simulink model "IEEE39_IBR_FrequencyControl_Primary_2022b"  (R2022b)
settings: Solver=VariableStepAuto  StartTime=0.0  StopTime=30  RelTol=1e-3
InitFcn:
  | IEEE39data_FrencyControl_primary;
undefined symbols (not defined in the file): Fref, IBR_data, line, Sbase, t_start_disturbance, Vbase
libraries: spsThreePhaseVIMeasurementLib x61, spsThreePhasePISectionLineLib x34, spsControlledVoltageSourceLib x33, spsabctodq0Lib x33, powerlib_extras x27, spsPLL3phLib x26, spsGroundLib x22, spsThreePhaseSeriesRLCBranchLib x22, spsThreePhaseParallelRLCLoadLib x20, slpidlib x14, spsMeanLib x11, spsdq0toabcLib x11
(part 3 of 5)

== system IEEE39_IBR_FrequencyControl_Primary_2022b/GFM4/PV_PQ3 ==
  Pref : Inport
  Vref_LL : Inport  Port=2
  Fref : Inport  Port=3
  Initial_phase : Inport  Port=4
  3-phase Instantaneous Active & Reactive Power4 : powerlib_extras/Measurements/3-phase  Instantaneous  Active & Reactive Power
  Controlled Voltage Source : spsControlledVoltageSourceLib/Controlled Voltage Source  Initialize=on  Source_Type=DC  Amplitude=0  Phase=0  Frequency=60  Measurements=None
  Controlled Voltage Source1 : spsControlledVoltageSourceLib/Controlled Voltage Source  Initialize=on  Source_Type=DC  Amplitude=0  Phase=-120  Frequency=60  Measurements=None
  Controlled Voltage Source3 : spsControlledVoltageSourceLib/Controlled Voltage Source  Initialize=on  Source_Type=DC  Amplitude=0  Phase=120  Frequency=60  Measurements=None
  Demux : Demux  Outputs=2
  Freq_Droop : Subsystem
  Ground : spsGroundLib/Ground  LConnTagsString=a
  Ground1 : spsGroundLib/Ground  LConnTagsString=a
  L : spsThreePhaseSeriesRLCBranchLib/Three-Phase Series RLC Branch  LConnTagsString=A|B|C  RConnTagsString=A|B|C  BranchType=L  Resistance=1  Inductance=0.01  Capacitance=1.0  Measurements=None
  Mean : spsMeanLib/Mean  Freq=60  Vinit=0  Ts=5e-4
  Three-Phase Series RLC Branch : spsThreePhaseSeriesRLCBranchLib/Three-Phase Series RLC Branch  LConnTagsString=A|B|C  RConnTagsString=A|B|C  BranchType=C  Resistance=0  Inductance=1e-3  Capacitance=1e-6  Measurements=None
  Three-Phase V-I Measurement : spsThreePhaseVIMeasurementLib/Three-Phase V-I Measurement  VoltageMeasurement=phase-to-ground  SetLabelV=off  LabelV=Vabc  Vpu=off  VpuLL=off  CurrentMeasurement=yes  SetLabelI=off  LabelI=Iabc  Ipu=off  Pbase=1e5  Vbase=380  OutputType=Complex  PhasorSimulation=off  PSBequivalent=0
  Three-Phase V-I Measurement4 : spsThreePhaseVIMeasurementLib/Three-Phase V-I Measurement  VoltageMeasurement=no  SetLabelV=off  LabelV=u  Vpu=off  VpuLL=off  CurrentMeasurement=yes  SetLabelI=off  LabelI=iFabcp3  Ipu=off  Pbase=100e6  Vbase=500e3  OutputType=Complex  PhasorSimulation=off  PSBequivalent=0
  Unit Delay : UnitDelay  SampleTime=-1  HasFrameUpgradeWarning=on
  Unit Delay1 : UnitDelay  SampleTime=-1  HasFrameUpgradeWarning=on
  Unit Delay2 : UnitDelay  SampleTime=-1  HasFrameUpgradeWarning=on
  V/F : Subsystem
  PV_BatteryA : PMIOPort  Side=Right
  PV_BatteryB : PMIOPort  Port=2  Side=Right
  PV_BatteryC : PMIOPort  Port=3  Side=Right
  tag scope: P_GFM7=global
  wires:
  Three-Phase V-I Measurement/1 -> 3-phase Instantaneous Active & Reactive Power4/1, V/F/1(vabcb)
  Three-Phase V-I Measurement/2 -> V/F/2(iabcb), 3-phase Instantaneous Active & Reactive Power4/2
  Mean/1 -> Demux/1
  3-phase Instantaneous Active & Reactive Power4/1 -> Mean/1
  Pref/1 -> Freq_Droop/1(Pref)
  Fref/1 -> Freq_Droop/2(Fref)
  [P_meas] -> Freq_Droop/3(Pmeans)
  Freq_Droop/1(fset) -> V/F/5(f)
  Vref_LL/1 -> V/F/4(Vref_LL)
  Initial_phase/1 -> V/F/6(Init_Phase_degree)
  Unit Delay/1 -> Controlled Voltage Source/1
  V/F/1(Va) -> Unit Delay/1
  Unit Delay1/1 -> Controlled Voltage Source1/1
  V/F/2(Vb) -> Unit Delay1/1
  Unit Delay2/1 -> Controlled Voltage Source3/1
  V/F/3(Vc) -> Unit Delay2/1
  Demux/1 -> [P_meas], [P_GFM7]
  Three-Phase V-I Measurement4/1 -> V/F/3(iFabcb)
  connections:
  Three-Phase V-I Measurement/RConn2 -- PV_BatteryB/RConn1
  Three-Phase V-I Measurement/LConn2 -- Three-Phase Series RLC Branch/LConn2 -- L/RConn2
  Three-Phase V-I Measurement4/LConn2 -- Controlled Voltage Source1/RConn1
  Controlled Voltage Source/RConn1 -- Three-Phase V-I Measurement4/LConn1
  Three-Phase V-I Measurement4/LConn3 -- Controlled Voltage Source3/RConn1
  Three-Phase V-I Measurement/LConn3 -- Three-Phase Series RLC Branch/LConn3 -- L/RConn3
  Three-Phase V-I Measurement/RConn3 -- PV_BatteryC/RConn1
  Three-Phase V-I Measurement/RConn1 -- PV_BatteryA/RConn1
  Three-Phase V-I Measurement4/RConn1 -- L/LConn1
  Three-Phase V-I Measurement4/RConn2 -- L/LConn2
  Three-Phase V-I Measurement4/RConn3 -- L/LConn3
  Three-Phase Series RLC Branch/RConn1 -- Ground1/LConn1 -- Three-Phase Series RLC Branch/RConn2 -- Three-Phase Series RLC Branch/RConn3
  Controlled Voltage Source/LConn1 -- Controlled Voltage Source3/LConn1 -- Controlled Voltage Source1/LConn1 -- Ground/LConn1
  Three-Phase V-I Measurement/LConn1 -- Three-Phase Series RLC Branch/LConn1 -- L/RConn1

== system IEEE39_IBR_FrequencyControl_Primary_2022b/PV/PV_PQ3 ==
  Pref : Inport
  Qref : Inport  Port=2
  3-phase Instantaneous Active & Reactive Power4 : powerlib_extras/Measurements/3-phase  Instantaneous  Active & Reactive Power
  Controlled Voltage Source : spsControlledVoltageSourceLib/Controlled Voltage Source  Initialize=on  Source_Type=AC  Amplitude=391.87  Phase=0  Frequency=60  Measurements=None
  Controlled Voltage Source1 : spsControlledVoltageSourceLib/Controlled Voltage Source  Initialize=on  Source_Type=AC  Amplitude=391.87  Phase=-120  Frequency=60  Measurements=None
  Controlled Voltage Source3 : spsControlledVoltageSourceLib/Controlled Voltage Source  Initialize=on  Source_Type=AC  Amplitude=391.87  Phase=120  Frequency=60  Measurements=None
  Demux : Demux  Outputs=2
  Ground : spsGroundLib/Ground  LConnTagsString=a
  Ground1 : spsGroundLib/Ground  LConnTagsString=a
  L : spsThreePhaseSeriesRLCBranchLib/Three-Phase Series RLC Branch  LConnTagsString=A|B|C  RConnTagsString=A|B|C  BranchType=RL  Resistance=0  Inductance=10e-3  Capacitance=1.0  Measurements=None
  L1 : Constant  Value=10e-3
  Mean : spsMeanLib/Mean  Freq=60  Vinit=0  Ts=5e-4
  PLL (3ph) : spsPLL3phLib/PLL (3ph)  Fmin=59.5  Par_Init=[0, 60]  ParK=[180, 3200, 1]  TcD=1e-4  MaxRateChangeFreq=12  FilterCutOffFreq=25  Ts=1e-5  AGC=on
  Scope1 : Scope
  Subsystem2 : Subsystem
  Terminator : Terminator
  Terminator1 : Terminator
  Three-Phase Series RLC Branch : spsThreePhaseSeriesRLCBranchLib/Three-Phase Series RLC Branch  LConnTagsString=A|B|C  RConnTagsString=A|B|C  BranchType=RC  Resistance=1000000  Inductance=1e-3  Capacitance=100e-6  Measurements=None
  Three-Phase V-I Measurement : spsThreePhaseVIMeasurementLib/Three-Phase V-I Measurement  VoltageMeasurement=phase-to-ground  SetLabelV=off  LabelV=Vabc  Vpu=off  VpuLL=off  CurrentMeasurement=yes  SetLabelI=off  LabelI=Iabc  Ipu=off  Pbase=1e5  Vbase=380  OutputType=Complex  PhasorSimulation=off  PSBequivalent=0
  Three-Phase V-I Measurement4 : spsThreePhaseVIMeasurementLib/Three-Phase V-I Measurement  VoltageMeasurement=no  SetLabelV=off  LabelV=u  Vpu=off  VpuLL=off  CurrentMeasurement=yes  SetLabelI=off  LabelI=iFabcp3  Ipu=off  Pbase=100e6  Vbase=500e3  OutputType=Complex  PhasorSimulation=off  PSBequivalent=0
  Unit Delay : UnitDelay  SampleTime=-1  HasFrameUpgradeWarning=on
  Unit Delay1 : UnitDelay  SampleTime=-1  HasFrameUpgradeWarning=on
  Unit Delay2 : UnitDelay  SampleTime=-1  HasFrameUpgradeWarning=on
  PV_BatteryA : PMIOPort  Side=Right
  PV_BatteryB : PMIOPort  Port=2  Side=Right
  PV_BatteryC : PMIOPort  Port=3  Side=Right
  wires:
  Three-Phase V-I Measurement/1 -> 3-phase Instantaneous Active & Reactive Power4/1, PLL (3ph)/1, Subsystem2/1(Vabcp)
  Three-Phase V-I Measurement/2 -> Subsystem2/2(Iabcp), 3-phase Instantaneous Active & Reactive Power4/2
  Mean/1 -> Demux/1
  L1/1 -> Subsystem2/6(L1)
  Three-Phase V-I Measurement4/1 -> Subsystem2/3(IFabcp)
  3-phase Instantaneous Active & Reactive Power4/1 -> Mean/1
  Qref/1 -> Subsystem2/5(Q_set)
  PLL (3ph)/1 -> [Freq]
  Pref/1 -> Subsystem2/4(P_set)
  Subsystem2/1(Va) -> Unit Delay/1
  Unit Delay/1 -> Controlled Voltage Source/1
  Subsystem2/2(Vb) -> Unit Delay1/1
  Unit Delay1/1 -> Controlled Voltage Source1/1
  Subsystem2/3(Vc) -> Unit Delay2/1
  Unit Delay2/1 -> Controlled Voltage Source3/1
  PLL (3ph)/2 -> Terminator/1
  Demux/2 -> Terminator1/1
  Demux/1 -> Scope1/1
  connections:
  Three-Phase V-I Measurement/LConn1 -- Three-Phase Series RLC Branch/LConn1 -- L/RConn1
  Three-Phase V-I Measurement/RConn2 -- PV_BatteryB/RConn1
  Three-Phase V-I Measurement/LConn2 -- Three-Phase Series RLC Branch/LConn2 -- L/RConn2
  Three-Phase V-I Measurement4/LConn2 -- Controlled Voltage Source1/RConn1
  Controlled Voltage Source/RConn1 -- Three-Phase V-I Measurement4/LConn1
  Three-Phase V-I Measurement4/LConn3 -- Controlled Voltage Source3/RConn1
  Three-Phase V-I Measurement/LConn3 -- Three-Phase Series RLC Branch/LConn3 -- L/RConn3
  Three-Phase V-I Measurement/RConn3 -- PV_BatteryC/RConn1
  Three-Phase V-I Measurement/RConn1 -- PV_BatteryA/RConn1
  Three-Phase V-I Measurement4/RConn1 -- L/LConn1
  Three-Phase V-I Measurement4/RConn2 -- L/LConn2
  Three-Phase V-I Measurement4/RConn3 -- L/LConn3
  Three-Phase Series RLC Branch/RConn1 -- Ground1/LConn1 -- Three-Phase Series RLC Branch/RConn2 -- Three-Phase Series RLC Branch/RConn3
  Controlled Voltage Source/LConn1 -- Controlled Voltage Source3/LConn1 -- Controlled Voltage Source1/LConn1 -- Ground/LConn1

== system IEEE39_IBR_FrequencyControl_Primary_2022b/G1_GFL/PV_PQ3/Freq_Droop ==
  Pref : Inport
  Fref : Inport  Port=2
  Freq : Inport  Port=3
  D : Inport  Port=4
  Divide : Product  Inputs=*/
  Product : Product
  Product1 : Product
  S_base : Constant  Value=Sbase
  Saturation : Saturate  UpperLimit=10*Sbase  LowerLimit=0  ZeroCross=off
  Sum : Sum  Inputs=|+-
  Sum1 : Sum  Inputs=|+-
  Transfer Fcn : TransferFcn  Denominator=[0.318 1]
  Pset : Outport
  wires:
  Freq/1 -> Sum/1
  Fref/1 -> Sum/2, Divide/2
  S_base/1 -> Product/2
  D/1 -> Product1/1
  Product/1 -> Product1/2
  Pref/1 -> Sum1/1
  Product1/1 -> Sum1/2
  Saturation/1 -> Pset/1
  Sum1/1 -> Saturation/1
  Sum/1 -> Divide/1
  Transfer Fcn/1 -> Product/1
  Divide/1 -> Transfer Fcn/1

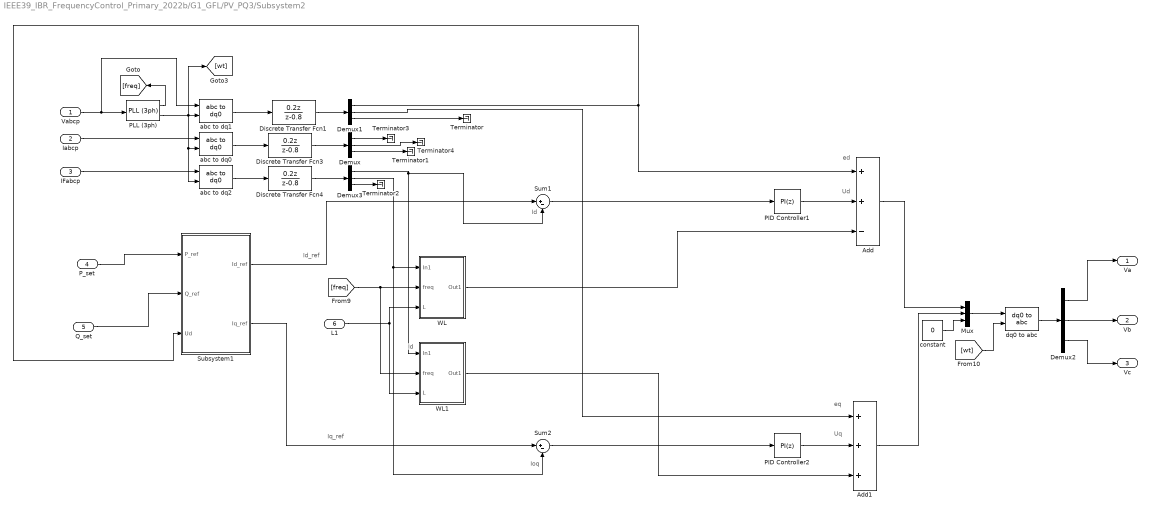
== system IEEE39_IBR_FrequencyControl_Primary_2022b/G1_GFL/PV_PQ3/Subsystem2 ==
  note: Iq_ref
  note: Id
  note: Id_ref
  note: Ud
  note: Uq
  note: eq
  note: ed
  note: Ioq
  note: Id
  Vabcp : Inport
  Iabcp : Inport  Port=2
  IFabcp : Inport  Port=3
  P_set : Inport  Port=4
  Q_set : Inport  Port=5
  L1 : Inport  Port=6
  Add : Sum  Inputs=++-
  Add1 : Sum  Inputs=+++
  Demux{,1..3} (4 alike) : Demux  Outputs=3
  Discrete Transfer Fcn1 : DiscreteTransferFcn  Numerator=[0.2 0]  Denominator=[1 -0.8]  InitialStates=[1 1 1]  SampleTime=5e-4
  Discrete Transfer Fcn3 : DiscreteTransferFcn  Numerator=[0.2 0]  Denominator=[1 -0.8]  SampleTime=5e-4
  Discrete Transfer Fcn4 : DiscreteTransferFcn  Numerator=[0.2 0]  Denominator=[1 -0.8]  SampleTime=5e-4
  Mux : Mux  Inputs=3
  PID Controller1 : slpidlib/PID Controller  Controller=PI  Form=Parallel  TimeDomain=Discrete-time  UseExternalTs=off  SampleTime=5e-4  IntegratorMethod=Forward Euler  FilterMethod=Forward Euler  ControllerParametersSource=internal  P=50  I=400  UseKiTs=off  D=0  N=100  UseFilter=on  TunerSelectOption=Transfer Function Based (PID Tuner App)  InitialConditionSource=internal  InitialConditionForIntegrator=0  InitialConditionForFilter=0  DifferentiatorICPrevScaledInput=0  ExternalReset=none  TrackingMode=off  Kt=1  LimitOutput=off  SatLimitsSource=internal  UpperSaturationLimit=inf  LowerSaturationLimit=-inf  LinearizeAsGain=on  AntiWindupMode=none  Kb=1  LimitIntegrator=off  UpperIntegratorSaturationLimit=inf  LowerIntegratorSaturationLimit=-inf  POutMin=[]  POutMax=[]  IOutMin=[]  IOutMax=[]  DOutMin=[]  DOutMax=[]  NOutMin=[]  NOutMax=[]  SumOutMin=[]  SumOutMax=[]  SaturationOutMin=[]  SaturationOutMax=[]  PParamMin=[]  PParamMax=[]  IParamMin=[]  IParamMax=[]  DParamMin=[]  DParamMax=[]  NParamMin=[]  NParamMax=[]  KbParamMin=[]  KbParamMax=[]  KtParamMin=[]  KtParamMax=[]  KbOutMin=[]  KbOutMax=[]  KtOutMin=[]  KtOutMax=[]  IntegratorOutMin=[]  IntegratorOutMax=[]  FilterOutMin=[]  FilterOutMax=[]  SumI1OutMin=[]  SumI1OutMax=[]  SumI2OutMin=[]  SumI2OutMax=[]  SumI3OutMin=[]  SumI3OutMax=[]  SumI4OutMin=[]  SumI4OutMax=[]  SumDOutMin=[]  SumDOutMax=[]  DifferentiatorOutMin=[]  DifferentiatorOutMax=[]  FilterDiffOutCoefMin=[]  FilterDiffOutCoefMax=[]  ReciprocalOutMin=[]  ReciprocalOutMax=[]  SumDenOutMin=[]  SumDenOutMax=[]  SumNumOutMin=[]  SumNumOutMax=[]  DivideOutMin=[]  DivideOutMax=[]  UdiffTsProdOutMin=[]  UdiffTsProdOutMax=[]  NTsProdOutMin=[]  NTsProdOutMax=[]  UintegralTsProdOutMin=[]  UintegralTsProdOutMax=[]  UngainTsProdOutMin=[]  UngainTsProdOutMax=[]  IntegratorContinuousStateAttributes=''  IntegratorStateMustResolveToSignalObject=off  IntegratorRTWStateStorageClass=Auto  FilterContinuousStateAttributes=''  FilterStateMustResolveToSignalObject=off  FilterRTWStateStorageClass=Auto  ParallelPVariant=InternalParameters  IdealPVariant=Disabled  IVariant=InternalParameters  DVariant=Disabled  IntegratorVariant=Discrete  SatVariant=Disabled  AWVariant=Passthrough  PCopyVariant=Disabled  TRVariant=Disabled  FdbkBlocksVariant=Forward  IdealPFdbkVariant=Disabled  SatFdbkVariant=Disabled  DerivativeFilterVariant=Disabled  NVariant=Disabled  NCopyVariant=Disabled_SignalSpec  FilterICVariant=Disabled  IntegratorICVariant=InternalICs  ExternalResetVariant=Disabled  TRSumVariant=Passthrough  SumFdbkVariant=Disabled  SumVariant=Sum_PI  TsampFilterVariant=InternalTs  TsampNgainVariant=Passthrough  TsampIntegralVariant=Disabled_SignalSpec  ExternalSaturationOutDataTypeStr=Inherit: Same as second input
  PID Controller2 : slpidlib/PID Controller  Controller=PI  Form=Parallel  TimeDomain=Discrete-time  UseExternalTs=off  SampleTime=5e-4  IntegratorMethod=Forward Euler  FilterMethod=Forward Euler  ControllerParametersSource=internal  P=50  I=400  UseKiTs=off  D=0  N=100  UseFilter=on  TunerSelectOption=Transfer Function Based (PID Tuner App)  InitialConditionSource=internal  InitialConditionForIntegrator=0  InitialConditionForFilter=0  DifferentiatorICPrevScaledInput=0  ExternalReset=none  TrackingMode=off  Kt=1  LimitOutput=off  SatLimitsSource=internal  UpperSaturationLimit=inf  LowerSaturationLimit=-inf  LinearizeAsGain=on  AntiWindupMode=none  Kb=1  LimitIntegrator=off  UpperIntegratorSaturationLimit=inf  LowerIntegratorSaturationLimit=-inf  POutMin=[]  POutMax=[]  IOutMin=[]  IOutMax=[]  DOutMin=[]  DOutMax=[]  NOutMin=[]  NOutMax=[]  SumOutMin=[]  SumOutMax=[]  SaturationOutMin=[]  SaturationOutMax=[]  PParamMin=[]  PParamMax=[]  IParamMin=[]  IParamMax=[]  DParamMin=[]  DParamMax=[]  NParamMin=[]  NParamMax=[]  KbParamMin=[]  KbParamMax=[]  KtParamMin=[]  KtParamMax=[]  KbOutMin=[]  KbOutMax=[]  KtOutMin=[]  KtOutMax=[]  IntegratorOutMin=[]  IntegratorOutMax=[]  FilterOutMin=[]  FilterOutMax=[]  SumI1OutMin=[]  SumI1OutMax=[]  SumI2OutMin=[]  SumI2OutMax=[]  SumI3OutMin=[]  SumI3OutMax=[]  SumI4OutMin=[]  SumI4OutMax=[]  SumDOutMin=[]  SumDOutMax=[]  DifferentiatorOutMin=[]  DifferentiatorOutMax=[]  FilterDiffOutCoefMin=[]  FilterDiffOutCoefMax=[]  ReciprocalOutMin=[]  ReciprocalOutMax=[]  SumDenOutMin=[]  SumDenOutMax=[]  SumNumOutMin=[]  SumNumOutMax=[]  DivideOutMin=[]  DivideOutMax=[]  UdiffTsProdOutMin=[]  UdiffTsProdOutMax=[]  NTsProdOutMin=[]  NTsProdOutMax=[]  UintegralTsProdOutMin=[]  UintegralTsProdOutMax=[]  UngainTsProdOutMin=[]  UngainTsProdOutMax=[]  IntegratorContinuousStateAttributes=''  IntegratorStateMustResolveToSignalObject=off  IntegratorRTWStateStorageClass=Auto  FilterContinuousStateAttributes=''  FilterStateMustResolveToSignalObject=off  FilterRTWStateStorageClass=Auto  ParallelPVariant=InternalParameters  IdealPVariant=Disabled  IVariant=InternalParameters  DVariant=Disabled  IntegratorVariant=Discrete  SatVariant=Disabled  AWVariant=Passthrough  PCopyVariant=Disabled  TRVariant=Disabled  FdbkBlocksVariant=Forward  IdealPFdbkVariant=Disabled  SatFdbkVariant=Disabled  DerivativeFilterVariant=Disabled  NVariant=Disabled  NCopyVariant=Disabled_SignalSpec  FilterICVariant=Disabled  IntegratorICVariant=InternalICs  ExternalResetVariant=Disabled  TRSumVariant=Passthrough  SumFdbkVariant=Disabled  SumVariant=Sum_PI  TsampFilterVariant=InternalTs  TsampNgainVariant=Passthrough  TsampIntegralVariant=Disabled_SignalSpec  ExternalSaturationOutDataTypeStr=Inherit: Same as second input
  PLL (3ph) : spsPLL3phLib/PLL (3ph)  Fmin=59.5  Par_Init=[0, 60]  ParK=[180, 3200, 1]  TcD=1e-4  MaxRateChangeFreq=12  FilterCutOffFreq=25  Ts=1e-5  AGC=on
  Subsystem1 : Subsystem
  Sum1 : Sum  Inputs=|+-
  Sum2 : Sum  Inputs=|+-
  Terminator{,1..4} (5 alike) : Terminator
  WL : Subsystem
  WL1 : Subsystem
  abc to dq0 : spsabctodq0Lib/abc to dq0  Alignment=90 degrees behind phase A axis
  abc to dq1 : spsabctodq0Lib/abc to dq0  Alignment=90 degrees behind phase A axis
  abc to dq2 : spsabctodq0Lib/abc to dq0  Alignment=90 degrees behind phase A axis
  constant : Constant  Value=0
  dq0 to abc : spsdq0toabcLib/dq0 to abc  Alignment=90 degrees behind phase A axis
  Va : Outport  VectorParamsAs1DForOutWhenUnconnected=off
  Vb : Outport  Port=2  VectorParamsAs1DForOutWhenUnconnected=off
  Vc : Outport  Port=3  VectorParamsAs1DForOutWhenUnconnected=off
  wires:
  abc to dq0/1 -> Discrete Transfer Fcn3/1
  PLL (3ph)/2 -> [wt], abc to dq1/2, abc to dq2/2, abc to dq0/2
  Demux1/1 -> Add/1, Subsystem1/3(Ud)
  L1/1 -> WL/3(L), WL1/3(L)
  WL/1(Out1) -> Add/3
  [freq] -> WL1/2(freq), WL/2(freq)
  PLL (3ph)/1 -> [freq]
  Demux2/1 -> Va/1
  Add/1 -> Mux/1
  PID Controller2/1 -> Add1/2
  Demux2/2 -> Vb/1
  WL1/1(Out1) -> Add1/3
  Demux1/2 -> Add1/1
  Add1/1 -> Mux/2
  Mux/1 -> dq0 to abc/1
  Demux2/3 -> Vc/1
  dq0 to abc/1 -> Demux2/1
  Subsystem1/1(Id_ref) -> Sum1/1
  PID Controller1/1 -> Add/2
  [wt] -> dq0 to abc/2
  Subsystem1/2(Iq_ref) -> Sum2/1
  Demux1/3 -> Terminator/1
  Demux/3 -> Terminator1/1
  constant/1 -> Mux/3
  IFabcp/1 -> abc to dq2/1
  abc to dq2/1 -> Discrete Transfer Fcn4/1
  Demux3/3 -> Terminator2/1
  Demux3/2 -> Sum2/2, WL/1(In1)
  Demux3/1 -> Sum1/2, WL1/1(In1)
  Sum1/1 -> PID Controller1/1
  Sum2/1 -> PID Controller2/1
  P_set/1 -> Subsystem1/1(P_ref)
  Q_set/1 -> Subsystem1/2(Q_ref)
  Discrete Transfer Fcn3/1 -> Demux/1
  Discrete Transfer Fcn4/1 -> Demux3/1
  Demux/1 -> Terminator3/1
  Demux/2 -> Terminator4/1
  Discrete Transfer Fcn1/1 -> Demux1/1
  Iabcp/1 -> abc to dq0/1
  Vabcp/1 -> abc to dq1/1, PLL (3ph)/1
  abc to dq1/1 -> Discrete Transfer Fcn1/1

== system IEEE39_IBR_FrequencyControl_Primary_2022b/G2_GFL/PV_PQ3/Freq_Droop ==
  Pref : Inport
  Fref : Inport  Port=2
  Freq : Inport  Port=3
  D : Inport  Port=4
  Divide : Product  Inputs=*/
  Product : Product
  Product1 : Product
  S_base : Constant  Value=Sbase
  Saturation : Saturate  UpperLimit=10*Sbase  LowerLimit=0  ZeroCross=off
  Sum : Sum  Inputs=|+-
  Sum1 : Sum  Inputs=|+-
  Transfer Fcn : TransferFcn  Denominator=[0.318 1]
  Pset : Outport
  wires:
  Freq/1 -> Sum/1
  Fref/1 -> Sum/2, Divide/2
  S_base/1 -> Product/2
  D/1 -> Product1/1
  Product/1 -> Product1/2
  Pref/1 -> Sum1/1
  Product1/1 -> Sum1/2
  Saturation/1 -> Pset/1
  Sum1/1 -> Saturation/1
  Sum/1 -> Divide/1
  Transfer Fcn/1 -> Product/1
  Divide/1 -> Transfer Fcn/1

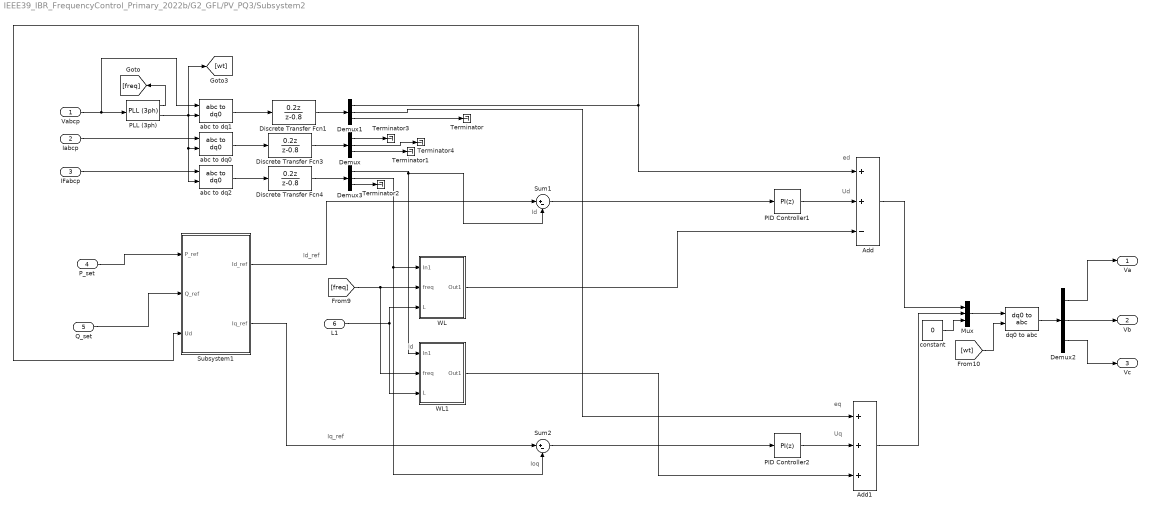
== system IEEE39_IBR_FrequencyControl_Primary_2022b/G2_GFL/PV_PQ3/Subsystem2 ==
  note: Iq_ref
  note: Id
  note: Id_ref
  note: Ud
  note: Uq
  note: eq
  note: ed
  note: Ioq
  note: Id
  Vabcp : Inport
  Iabcp : Inport  Port=2
  IFabcp : Inport  Port=3
  P_set : Inport  Port=4
  Q_set : Inport  Port=5
  L1 : Inport  Port=6
  Add : Sum  Inputs=++-
  Add1 : Sum  Inputs=+++
  Demux{,1..3} (4 alike) : Demux  Outputs=3
  Discrete Transfer Fcn1 : DiscreteTransferFcn  Numerator=[0.2 0]  Denominator=[1 -0.8]  InitialStates=[1 1 1]  SampleTime=5e-4
  Discrete Transfer Fcn3 : DiscreteTransferFcn  Numerator=[0.2 0]  Denominator=[1 -0.8]  SampleTime=5e-4
  Discrete Transfer Fcn4 : DiscreteTransferFcn  Numerator=[0.2 0]  Denominator=[1 -0.8]  SampleTime=5e-4
  Mux : Mux  Inputs=3
  PID Controller1 : slpidlib/PID Controller  Controller=PI  Form=Parallel  TimeDomain=Discrete-time  UseExternalTs=off  SampleTime=5e-4  IntegratorMethod=Forward Euler  FilterMethod=Forward Euler  ControllerParametersSource=internal  P=50  I=400  UseKiTs=off  D=0  N=100  UseFilter=on  TunerSelectOption=Transfer Function Based (PID Tuner App)  InitialConditionSource=internal  InitialConditionForIntegrator=0  InitialConditionForFilter=0  DifferentiatorICPrevScaledInput=0  ExternalReset=none  TrackingMode=off  Kt=1  LimitOutput=off  SatLimitsSource=internal  UpperSaturationLimit=inf  LowerSaturationLimit=-inf  LinearizeAsGain=on  AntiWindupMode=none  Kb=1  LimitIntegrator=off  UpperIntegratorSaturationLimit=inf  LowerIntegratorSaturationLimit=-inf  POutMin=[]  POutMax=[]  IOutMin=[]  IOutMax=[]  DOutMin=[]  DOutMax=[]  NOutMin=[]  NOutMax=[]  SumOutMin=[]  SumOutMax=[]  SaturationOutMin=[]  SaturationOutMax=[]  PParamMin=[]  PParamMax=[]  IParamMin=[]  IParamMax=[]  DParamMin=[]  DParamMax=[]  NParamMin=[]  NParamMax=[]  KbParamMin=[]  KbParamMax=[]  KtParamMin=[]  KtParamMax=[]  KbOutMin=[]  KbOutMax=[]  KtOutMin=[]  KtOutMax=[]  IntegratorOutMin=[]  IntegratorOutMax=[]  FilterOutMin=[]  FilterOutMax=[]  SumI1OutMin=[]  SumI1OutMax=[]  SumI2OutMin=[]  SumI2OutMax=[]  SumI3OutMin=[]  SumI3OutMax=[]  SumI4OutMin=[]  SumI4OutMax=[]  SumDOutMin=[]  SumDOutMax=[]  DifferentiatorOutMin=[]  DifferentiatorOutMax=[]  FilterDiffOutCoefMin=[]  FilterDiffOutCoefMax=[]  ReciprocalOutMin=[]  ReciprocalOutMax=[]  SumDenOutMin=[]  SumDenOutMax=[]  SumNumOutMin=[]  SumNumOutMax=[]  DivideOutMin=[]  DivideOutMax=[]  UdiffTsProdOutMin=[]  UdiffTsProdOutMax=[]  NTsProdOutMin=[]  NTsProdOutMax=[]  UintegralTsProdOutMin=[]  UintegralTsProdOutMax=[]  UngainTsProdOutMin=[]  UngainTsProdOutMax=[]  IntegratorContinuousStateAttributes=''  IntegratorStateMustResolveToSignalObject=off  IntegratorRTWStateStorageClass=Auto  FilterContinuousStateAttributes=''  FilterStateMustResolveToSignalObject=off  FilterRTWStateStorageClass=Auto  ParallelPVariant=InternalParameters  IdealPVariant=Disabled  IVariant=InternalParameters  DVariant=Disabled  IntegratorVariant=Discrete  SatVariant=Disabled  AWVariant=Passthrough  PCopyVariant=Disabled  TRVariant=Disabled  FdbkBlocksVariant=Forward  IdealPFdbkVariant=Disabled  SatFdbkVariant=Disabled  DerivativeFilterVariant=Disabled  NVariant=Disabled  NCopyVariant=Disabled_SignalSpec  FilterICVariant=Disabled  IntegratorICVariant=InternalICs  ExternalResetVariant=Disabled  TRSumVariant=Passthrough  SumFdbkVariant=Disabled  SumVariant=Sum_PI  TsampFilterVariant=InternalTs  TsampNgainVariant=Passthrough  TsampIntegralVariant=Disabled_SignalSpec  ExternalSaturationOutDataTypeStr=Inherit: Same as second input
  PID Controller2 : slpidlib/PID Controller  Controller=PI  Form=Parallel  TimeDomain=Discrete-time  UseExternalTs=off  SampleTime=5e-4  IntegratorMethod=Forward Euler  FilterMethod=Forward Euler  ControllerParametersSource=internal  P=50  I=400  UseKiTs=off  D=0  N=100  UseFilter=on  TunerSelectOption=Transfer Function Based (PID Tuner App)  InitialConditionSource=internal  InitialConditionForIntegrator=0  InitialConditionForFilter=0  DifferentiatorICPrevScaledInput=0  ExternalReset=none  TrackingMode=off  Kt=1  LimitOutput=off  SatLimitsSource=internal  UpperSaturationLimit=inf  LowerSaturationLimit=-inf  LinearizeAsGain=on  AntiWindupMode=none  Kb=1  LimitIntegrator=off  UpperIntegratorSaturationLimit=inf  LowerIntegratorSaturationLimit=-inf  POutMin=[]  POutMax=[]  IOutMin=[]  IOutMax=[]  DOutMin=[]  DOutMax=[]  NOutMin=[]  NOutMax=[]  SumOutMin=[]  SumOutMax=[]  SaturationOutMin=[]  SaturationOutMax=[]  PParamMin=[]  PParamMax=[]  IParamMin=[]  IParamMax=[]  DParamMin=[]  DParamMax=[]  NParamMin=[]  NParamMax=[]  KbParamMin=[]  KbParamMax=[]  KtParamMin=[]  KtParamMax=[]  KbOutMin=[]  KbOutMax=[]  KtOutMin=[]  KtOutMax=[]  IntegratorOutMin=[]  IntegratorOutMax=[]  FilterOutMin=[]  FilterOutMax=[]  SumI1OutMin=[]  SumI1OutMax=[]  SumI2OutMin=[]  SumI2OutMax=[]  SumI3OutMin=[]  SumI3OutMax=[]  SumI4OutMin=[]  SumI4OutMax=[]  SumDOutMin=[]  SumDOutMax=[]  DifferentiatorOutMin=[]  DifferentiatorOutMax=[]  FilterDiffOutCoefMin=[]  FilterDiffOutCoefMax=[]  ReciprocalOutMin=[]  ReciprocalOutMax=[]  SumDenOutMin=[]  SumDenOutMax=[]  SumNumOutMin=[]  SumNumOutMax=[]  DivideOutMin=[]  DivideOutMax=[]  UdiffTsProdOutMin=[]  UdiffTsProdOutMax=[]  NTsProdOutMin=[]  NTsProdOutMax=[]  UintegralTsProdOutMin=[]  UintegralTsProdOutMax=[]  UngainTsProdOutMin=[]  UngainTsProdOutMax=[]  IntegratorContinuousStateAttributes=''  IntegratorStateMustResolveToSignalObject=off  IntegratorRTWStateStorageClass=Auto  FilterContinuousStateAttributes=''  FilterStateMustResolveToSignalObject=off  FilterRTWStateStorageClass=Auto  ParallelPVariant=InternalParameters  IdealPVariant=Disabled  IVariant=InternalParameters  DVariant=Disabled  IntegratorVariant=Discrete  SatVariant=Disabled  AWVariant=Passthrough  PCopyVariant=Disabled  TRVariant=Disabled  FdbkBlocksVariant=Forward  IdealPFdbkVariant=Disabled  SatFdbkVariant=Disabled  DerivativeFilterVariant=Disabled  NVariant=Disabled  NCopyVariant=Disabled_SignalSpec  FilterICVariant=Disabled  IntegratorICVariant=InternalICs  ExternalResetVariant=Disabled  TRSumVariant=Passthrough  SumFdbkVariant=Disabled  SumVariant=Sum_PI  TsampFilterVariant=InternalTs  TsampNgainVariant=Passthrough  TsampIntegralVariant=Disabled_SignalSpec  ExternalSaturationOutDataTypeStr=Inherit: Same as second input
  PLL (3ph) : spsPLL3phLib/PLL (3ph)  Fmin=59.5  Par_Init=[0, 60]  ParK=[180, 3200, 1]  TcD=1e-4  MaxRateChangeFreq=12  FilterCutOffFreq=25  Ts=1e-5  AGC=on
  Subsystem1 : Subsystem
  Sum1 : Sum  Inputs=|+-
  Sum2 : Sum  Inputs=|+-
  Terminator{,1..4} (5 alike) : Terminator
  WL : Subsystem
  WL1 : Subsystem
  abc to dq0 : spsabctodq0Lib/abc to dq0  Alignment=90 degrees behind phase A axis
  abc to dq1 : spsabctodq0Lib/abc to dq0  Alignment=90 degrees behind phase A axis
  abc to dq2 : spsabctodq0Lib/abc to dq0  Alignment=90 degrees behind phase A axis
  constant : Constant  Value=0
  dq0 to abc : spsdq0toabcLib/dq0 to abc  Alignment=90 degrees behind phase A axis
  Va : Outport  VectorParamsAs1DForOutWhenUnconnected=off
  Vb : Outport  Port=2  VectorParamsAs1DForOutWhenUnconnected=off
  Vc : Outport  Port=3  VectorParamsAs1DForOutWhenUnconnected=off
  wires:
  abc to dq0/1 -> Discrete Transfer Fcn3/1
  PLL (3ph)/2 -> [wt], abc to dq1/2, abc to dq2/2, abc to dq0/2
  Demux1/1 -> Add/1, Subsystem1/3(Ud)
  L1/1 -> WL/3(L), WL1/3(L)
  WL/1(Out1) -> Add/3
  [freq] -> WL1/2(freq), WL/2(freq)
  PLL (3ph)/1 -> [freq]
  Demux2/1 -> Va/1
  Add/1 -> Mux/1
  PID Controller2/1 -> Add1/2
  Demux2/2 -> Vb/1
  WL1/1(Out1) -> Add1/3
  Demux1/2 -> Add1/1
  Add1/1 -> Mux/2
  Mux/1 -> dq0 to abc/1
  Demux2/3 -> Vc/1
  dq0 to abc/1 -> Demux2/1
  Subsystem1/1(Id_ref) -> Sum1/1
  PID Controller1/1 -> Add/2
  [wt] -> dq0 to abc/2
  Subsystem1/2(Iq_ref) -> Sum2/1
  Demux1/3 -> Terminator/1
  Demux/3 -> Terminator1/1
  constant/1 -> Mux/3
  IFabcp/1 -> abc to dq2/1
  abc to dq2/1 -> Discrete Transfer Fcn4/1
  Demux3/3 -> Terminator2/1
  Demux3/2 -> Sum2/2, WL/1(In1)
  Demux3/1 -> Sum1/2, WL1/1(In1)
  Sum1/1 -> PID Controller1/1
  Sum2/1 -> PID Controller2/1
  P_set/1 -> Subsystem1/1(P_ref)
  Q_set/1 -> Subsystem1/2(Q_ref)
  Discrete Transfer Fcn3/1 -> Demux/1
  Discrete Transfer Fcn4/1 -> Demux3/1
  Demux/1 -> Terminator3/1
  Demux/2 -> Terminator4/1
  Discrete Transfer Fcn1/1 -> Demux1/1
  Iabcp/1 -> abc to dq0/1
  Vabcp/1 -> abc to dq1/1, PLL (3ph)/1
  abc to dq1/1 -> Discrete Transfer Fcn1/1

== system IEEE39_IBR_FrequencyControl_Primary_2022b/G3_GFL/PV_PQ3/Freq_Droop ==
  Pref : Inport
  Fref : Inport  Port=2
  Freq : Inport  Port=3
  D : Inport  Port=4
  Divide : Product  Inputs=*/
  Product : Product
  Product1 : Product
  S_base : Constant  Value=Sbase
  Saturation : Saturate  UpperLimit=10*Sbase  LowerLimit=0  ZeroCross=off
  Sum : Sum  Inputs=|+-
  Sum1 : Sum  Inputs=|+-
  Transfer Fcn : TransferFcn  Denominator=[0.318 1]
  Pset : Outport
  wires:
  Freq/1 -> Sum/1
  Fref/1 -> Sum/2, Divide/2
  S_base/1 -> Product/2
  D/1 -> Product1/1
  Product/1 -> Product1/2
  Pref/1 -> Sum1/1
  Product1/1 -> Sum1/2
  Saturation/1 -> Pset/1
  Sum1/1 -> Saturation/1
  Sum/1 -> Divide/1
  Transfer Fcn/1 -> Product/1
  Divide/1 -> Transfer Fcn/1

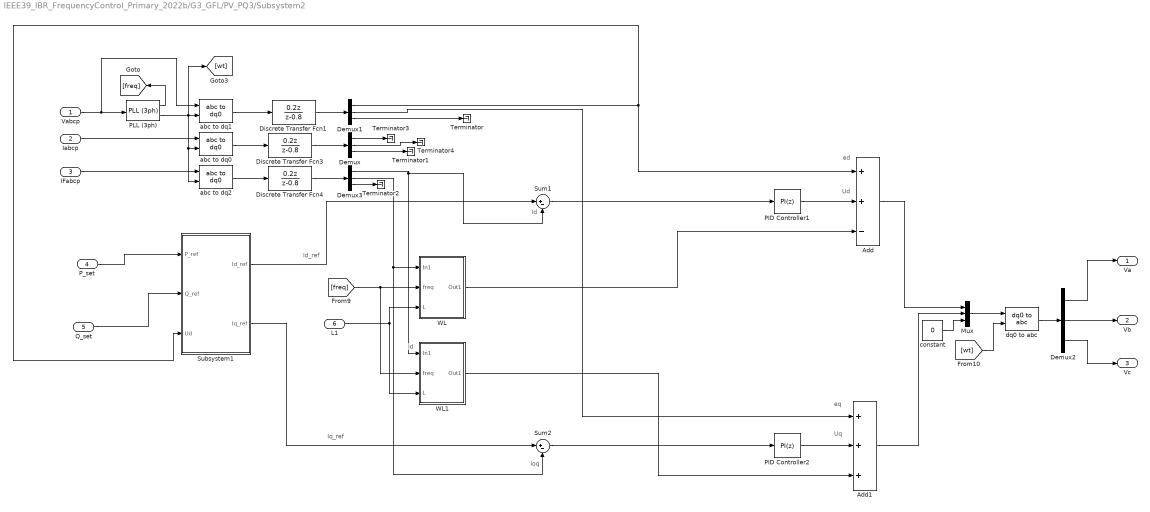
== system IEEE39_IBR_FrequencyControl_Primary_2022b/G3_GFL/PV_PQ3/Subsystem2 ==
  note: Iq_ref
  note: Id
  note: Id_ref
  note: Ud
  note: Uq
  note: eq
  note: ed
  note: Ioq
  note: Id
  Vabcp : Inport
  Iabcp : Inport  Port=2
  IFabcp : Inport  Port=3
  P_set : Inport  Port=4
  Q_set : Inport  Port=5
  L1 : Inport  Port=6
  Add : Sum  Inputs=++-
  Add1 : Sum  Inputs=+++
  Demux{,1..3} (4 alike) : Demux  Outputs=3
  Discrete Transfer Fcn1 : DiscreteTransferFcn  Numerator=[0.2 0]  Denominator=[1 -0.8]  InitialStates=[1 1 1]  SampleTime=5e-4
  Discrete Transfer Fcn3 : DiscreteTransferFcn  Numerator=[0.2 0]  Denominator=[1 -0.8]  SampleTime=5e-4
  Discrete Transfer Fcn4 : DiscreteTransferFcn  Numerator=[0.2 0]  Denominator=[1 -0.8]  SampleTime=5e-4
  Mux : Mux  Inputs=3
  PID Controller1 : slpidlib/PID Controller  Controller=PI  Form=Parallel  TimeDomain=Discrete-time  UseExternalTs=off  SampleTime=5e-4  IntegratorMethod=Forward Euler  FilterMethod=Forward Euler  ControllerParametersSource=internal  P=10  I=100  UseKiTs=off  D=0  N=100  UseFilter=on  TunerSelectOption=Transfer Function Based (PID Tuner App)  InitialConditionSource=internal  InitialConditionForIntegrator=0  InitialConditionForFilter=0  DifferentiatorICPrevScaledInput=0  ExternalReset=none  TrackingMode=off  Kt=1  LimitOutput=off  SatLimitsSource=internal  UpperSaturationLimit=inf  LowerSaturationLimit=-inf  LinearizeAsGain=on  AntiWindupMode=none  Kb=1  LimitIntegrator=off  UpperIntegratorSaturationLimit=inf  LowerIntegratorSaturationLimit=-inf  POutMin=[]  POutMax=[]  IOutMin=[]  IOutMax=[]  DOutMin=[]  DOutMax=[]  NOutMin=[]  NOutMax=[]  SumOutMin=[]  SumOutMax=[]  SaturationOutMin=[]  SaturationOutMax=[]  PParamMin=[]  PParamMax=[]  IParamMin=[]  IParamMax=[]  DParamMin=[]  DParamMax=[]  NParamMin=[]  NParamMax=[]  KbParamMin=[]  KbParamMax=[]  KtParamMin=[]  KtParamMax=[]  KbOutMin=[]  KbOutMax=[]  KtOutMin=[]  KtOutMax=[]  IntegratorOutMin=[]  IntegratorOutMax=[]  FilterOutMin=[]  FilterOutMax=[]  SumI1OutMin=[]  SumI1OutMax=[]  SumI2OutMin=[]  SumI2OutMax=[]  SumI3OutMin=[]  SumI3OutMax=[]  SumI4OutMin=[]  SumI4OutMax=[]  SumDOutMin=[]  SumDOutMax=[]  DifferentiatorOutMin=[]  DifferentiatorOutMax=[]  FilterDiffOutCoefMin=[]  FilterDiffOutCoefMax=[]  ReciprocalOutMin=[]  ReciprocalOutMax=[]  SumDenOutMin=[]  SumDenOutMax=[]  SumNumOutMin=[]  SumNumOutMax=[]  DivideOutMin=[]  DivideOutMax=[]  UdiffTsProdOutMin=[]  UdiffTsProdOutMax=[]  NTsProdOutMin=[]  NTsProdOutMax=[]  UintegralTsProdOutMin=[]  UintegralTsProdOutMax=[]  UngainTsProdOutMin=[]  UngainTsProdOutMax=[]  IntegratorContinuousStateAttributes=''  IntegratorStateMustResolveToSignalObject=off  IntegratorRTWStateStorageClass=Auto  FilterContinuousStateAttributes=''  FilterStateMustResolveToSignalObject=off  FilterRTWStateStorageClass=Auto  ParallelPVariant=InternalParameters  IdealPVariant=Disabled  IVariant=InternalParameters  DVariant=Disabled  IntegratorVariant=Discrete  SatVariant=Disabled  AWVariant=Passthrough  PCopyVariant=Disabled  TRVariant=Disabled  FdbkBlocksVariant=Forward  IdealPFdbkVariant=Disabled  SatFdbkVariant=Disabled  DerivativeFilterVariant=Disabled  NVariant=Disabled  NCopyVariant=Disabled_SignalSpec  FilterICVariant=Disabled  IntegratorICVariant=InternalICs  ExternalResetVariant=Disabled  TRSumVariant=Passthrough  SumFdbkVariant=Disabled  SumVariant=Sum_PI  TsampFilterVariant=InternalTs  TsampNgainVariant=Passthrough  TsampIntegralVariant=Disabled_SignalSpec  ExternalSaturationOutDataTypeStr=Inherit: Same as second input
  PID Controller2 : slpidlib/PID Controller  Controller=PI  Form=Parallel  TimeDomain=Discrete-time  UseExternalTs=off  SampleTime=5e-4  IntegratorMethod=Forward Euler  FilterMethod=Forward Euler  ControllerParametersSource=internal  P=10  I=100  UseKiTs=off  D=0  N=100  UseFilter=on  TunerSelectOption=Transfer Function Based (PID Tuner App)  InitialConditionSource=internal  InitialConditionForIntegrator=0  InitialConditionForFilter=0  DifferentiatorICPrevScaledInput=0  ExternalReset=none  TrackingMode=off  Kt=1  LimitOutput=off  SatLimitsSource=internal  UpperSaturationLimit=inf  LowerSaturationLimit=-inf  LinearizeAsGain=on  AntiWindupMode=none  Kb=1  LimitIntegrator=off  UpperIntegratorSaturationLimit=inf  LowerIntegratorSaturationLimit=-inf  POutMin=[]  POutMax=[]  IOutMin=[]  IOutMax=[]  DOutMin=[]  DOutMax=[]  NOutMin=[]  NOutMax=[]  SumOutMin=[]  SumOutMax=[]  SaturationOutMin=[]  SaturationOutMax=[]  PParamMin=[]  PParamMax=[]  IParamMin=[]  IParamMax=[]  DParamMin=[]  DParamMax=[]  NParamMin=[]  NParamMax=[]  KbParamMin=[]  KbParamMax=[]  KtParamMin=[]  KtParamMax=[]  KbOutMin=[]  KbOutMax=[]  KtOutMin=[]  KtOutMax=[]  IntegratorOutMin=[]  IntegratorOutMax=[]  FilterOutMin=[]  FilterOutMax=[]  SumI1OutMin=[]  SumI1OutMax=[]  SumI2OutMin=[]  SumI2OutMax=[]  SumI3OutMin=[]  SumI3OutMax=[]  SumI4OutMin=[]  SumI4OutMax=[]  SumDOutMin=[]  SumDOutMax=[]  DifferentiatorOutMin=[]  DifferentiatorOutMax=[]  FilterDiffOutCoefMin=[]  FilterDiffOutCoefMax=[]  ReciprocalOutMin=[]  ReciprocalOutMax=[]  SumDenOutMin=[]  SumDenOutMax=[]  SumNumOutMin=[]  SumNumOutMax=[]  DivideOutMin=[]  DivideOutMax=[]  UdiffTsProdOutMin=[]  UdiffTsProdOutMax=[]  NTsProdOutMin=[]  NTsProdOutMax=[]  UintegralTsProdOutMin=[]  UintegralTsProdOutMax=[]  UngainTsProdOutMin=[]  UngainTsProdOutMax=[]  IntegratorContinuousStateAttributes=''  IntegratorStateMustResolveToSignalObject=off  IntegratorRTWStateStorageClass=Auto  FilterContinuousStateAttributes=''  FilterStateMustResolveToSignalObject=off  FilterRTWStateStorageClass=Auto  ParallelPVariant=InternalParameters  IdealPVariant=Disabled  IVariant=InternalParameters  DVariant=Disabled  IntegratorVariant=Discrete  SatVariant=Disabled  AWVariant=Passthrough  PCopyVariant=Disabled  TRVariant=Disabled  FdbkBlocksVariant=Forward  IdealPFdbkVariant=Disabled  SatFdbkVariant=Disabled  DerivativeFilterVariant=Disabled  NVariant=Disabled  NCopyVariant=Disabled_SignalSpec  FilterICVariant=Disabled  IntegratorICVariant=InternalICs  ExternalResetVariant=Disabled  TRSumVariant=Passthrough  SumFdbkVariant=Disabled  SumVariant=Sum_PI  TsampFilterVariant=InternalTs  TsampNgainVariant=Passthrough  TsampIntegralVariant=Disabled_SignalSpec  ExternalSaturationOutDataTypeStr=Inherit: Same as second input
  PLL (3ph) : spsPLL3phLib/PLL (3ph)  Fmin=59.5  Par_Init=[0, 60]  ParK=[180, 3200, 1]  TcD=1e-4  MaxRateChangeFreq=12  FilterCutOffFreq=25  Ts=1e-5  AGC=on
  Subsystem1 : Subsystem
  Sum1 : Sum  Inputs=|+-
  Sum2 : Sum  Inputs=|+-
  Terminator{,1..4} (5 alike) : Terminator
  WL : Subsystem
  WL1 : Subsystem
  abc to dq0 : spsabctodq0Lib/abc to dq0  Alignment=90 degrees behind phase A axis
  abc to dq1 : spsabctodq0Lib/abc to dq0  Alignment=90 degrees behind phase A axis
  abc to dq2 : spsabctodq0Lib/abc to dq0  Alignment=90 degrees behind phase A axis
  constant : Constant  Value=0
  dq0 to abc : spsdq0toabcLib/dq0 to abc  Alignment=90 degrees behind phase A axis
  Va : Outport  VectorParamsAs1DForOutWhenUnconnected=off
  Vb : Outport  Port=2  VectorParamsAs1DForOutWhenUnconnected=off
  Vc : Outport  Port=3  VectorParamsAs1DForOutWhenUnconnected=off
  wires:
  abc to dq0/1 -> Discrete Transfer Fcn3/1
  PLL (3ph)/2 -> [wt], abc to dq1/2, abc to dq2/2, abc to dq0/2
  Demux1/1 -> Add/1, Subsystem1/3(Ud)
  L1/1 -> WL/3(L), WL1/3(L)
  WL/1(Out1) -> Add/3
  [freq] -> WL1/2(freq), WL/2(freq)
  PLL (3ph)/1 -> [freq]
  Demux2/1 -> Va/1
  Add/1 -> Mux/1
  PID Controller2/1 -> Add1/2
  Demux2/2 -> Vb/1
  WL1/1(Out1) -> Add1/3
  Demux1/2 -> Add1/1
  Add1/1 -> Mux/2
  Mux/1 -> dq0 to abc/1
  Demux2/3 -> Vc/1
  dq0 to abc/1 -> Demux2/1
  Subsystem1/1(Id_ref) -> Sum1/1
  PID Controller1/1 -> Add/2
  [wt] -> dq0 to abc/2
  Subsystem1/2(Iq_ref) -> Sum2/1
  Demux1/3 -> Terminator/1
  Demux/3 -> Terminator1/1
  constant/1 -> Mux/3
  IFabcp/1 -> abc to dq2/1
  abc to dq2/1 -> Discrete Transfer Fcn4/1
  Demux3/3 -> Terminator2/1
  Demux3/2 -> Sum2/2, WL/1(In1)
  Demux3/1 -> Sum1/2, WL1/1(In1)
  Sum1/1 -> PID Controller1/1
  Sum2/1 -> PID Controller2/1
  P_set/1 -> Subsystem1/1(P_ref)
  Q_set/1 -> Subsystem1/2(Q_ref)
  Discrete Transfer Fcn3/1 -> Demux/1
  Discrete Transfer Fcn4/1 -> Demux3/1
  Demux/1 -> Terminator3/1
  Demux/2 -> Terminator4/1
  Discrete Transfer Fcn1/1 -> Demux1/1
  Iabcp/1 -> abc to dq0/1
  Vabcp/1 -> abc to dq1/1, PLL (3ph)/1
  abc to dq1/1 -> Discrete Transfer Fcn1/1

== system IEEE39_IBR_FrequencyControl_Primary_2022b/G4_GFL1/PV_PQ3/Freq_Droop ==
  Pref : Inport
  Fref : Inport  Port=2
  Freq : Inport  Port=3
  D : Inport  Port=4
  Divide : Product  Inputs=*/
  Product : Product
  Product1 : Product
  S_base : Constant  Value=Sbase
  Saturation : Saturate  UpperLimit=10*Sbase  LowerLimit=0  ZeroCross=off
  Sum : Sum  Inputs=|+-
  Sum1 : Sum  Inputs=|+-
  Transfer Fcn : TransferFcn  Denominator=[0.318 1]
  Pset : Outport
  wires:
  Freq/1 -> Sum/1
  Fref/1 -> Sum/2, Divide/2
  S_base/1 -> Product/2
  D/1 -> Product1/1
  Product/1 -> Product1/2
  Pref/1 -> Sum1/1
  Product1/1 -> Sum1/2
  Saturation/1 -> Pset/1
  Sum1/1 -> Saturation/1
  Sum/1 -> Divide/1
  Transfer Fcn/1 -> Product/1
  Divide/1 -> Transfer Fcn/1

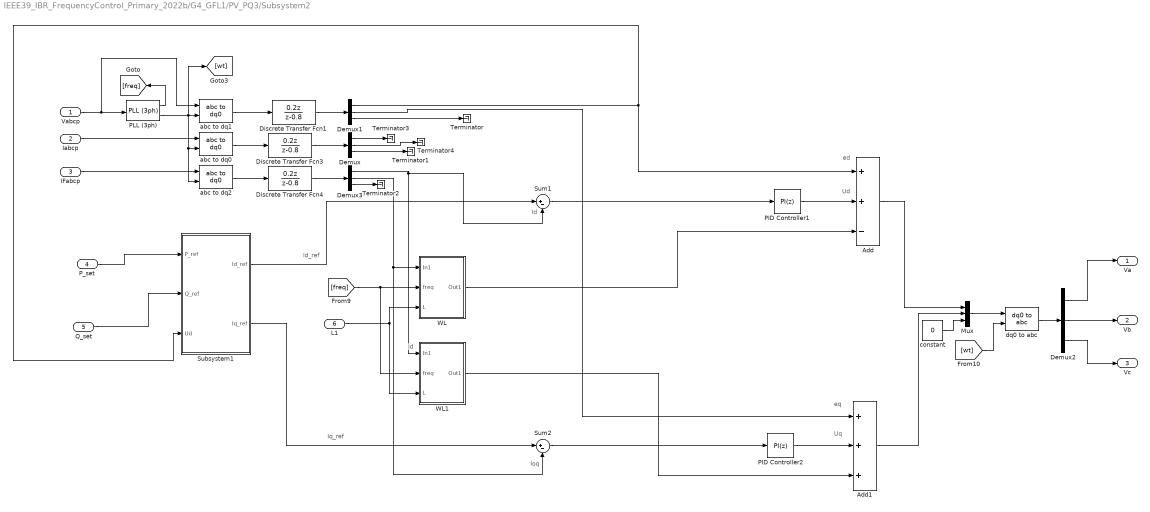
== system IEEE39_IBR_FrequencyControl_Primary_2022b/G4_GFL1/PV_PQ3/Subsystem2 ==
  note: Iq_ref
  note: Id
  note: Id_ref
  note: Ud
  note: Uq
  note: eq
  note: ed
  note: Ioq
  note: Id
  Vabcp : Inport
  Iabcp : Inport  Port=2
  IFabcp : Inport  Port=3
  P_set : Inport  Port=4
  Q_set : Inport  Port=5
  L1 : Inport  Port=6
  Add : Sum  Inputs=++-
  Add1 : Sum  Inputs=+++
  Demux{,1..3} (4 alike) : Demux  Outputs=3
  Discrete Transfer Fcn1 : DiscreteTransferFcn  Numerator=[0.2 0]  Denominator=[1 -0.8]  InitialStates=[1 1 1]  SampleTime=5e-4
  Discrete Transfer Fcn3 : DiscreteTransferFcn  Numerator=[0.2 0]  Denominator=[1 -0.8]  SampleTime=5e-4
  Discrete Transfer Fcn4 : DiscreteTransferFcn  Numerator=[0.2 0]  Denominator=[1 -0.8]  SampleTime=5e-4
  Mux : Mux  Inputs=3
  PID Controller1 : slpidlib/PID Controller  Controller=PI  Form=Parallel  TimeDomain=Discrete-time  UseExternalTs=off  SampleTime=5e-4  IntegratorMethod=Forward Euler  FilterMethod=Forward Euler  ControllerParametersSource=internal  P=50  I=400  UseKiTs=off  D=0  N=100  UseFilter=on  TunerSelectOption=Transfer Function Based (PID Tuner App)  InitialConditionSource=internal  InitialConditionForIntegrator=0  InitialConditionForFilter=0  DifferentiatorICPrevScaledInput=0  ExternalReset=none  TrackingMode=off  Kt=1  LimitOutput=off  SatLimitsSource=internal  UpperSaturationLimit=inf  LowerSaturationLimit=-inf  LinearizeAsGain=on  AntiWindupMode=none  Kb=1  LimitIntegrator=off  UpperIntegratorSaturationLimit=inf  LowerIntegratorSaturationLimit=-inf  POutMin=[]  POutMax=[]  IOutMin=[]  IOutMax=[]  DOutMin=[]  DOutMax=[]  NOutMin=[]  NOutMax=[]  SumOutMin=[]  SumOutMax=[]  SaturationOutMin=[]  SaturationOutMax=[]  PParamMin=[]  PParamMax=[]  IParamMin=[]  IParamMax=[]  DParamMin=[]  DParamMax=[]  NParamMin=[]  NParamMax=[]  KbParamMin=[]  KbParamMax=[]  KtParamMin=[]  KtParamMax=[]  KbOutMin=[]  KbOutMax=[]  KtOutMin=[]  KtOutMax=[]  IntegratorOutMin=[]  IntegratorOutMax=[]  FilterOutMin=[]  FilterOutMax=[]  SumI1OutMin=[]  SumI1OutMax=[]  SumI2OutMin=[]  SumI2OutMax=[]  SumI3OutMin=[]  SumI3OutMax=[]  SumI4OutMin=[]  SumI4OutMax=[]  SumDOutMin=[]  SumDOutMax=[]  DifferentiatorOutMin=[]  DifferentiatorOutMax=[]  FilterDiffOutCoefMin=[]  FilterDiffOutCoefMax=[]  ReciprocalOutMin=[]  ReciprocalOutMax=[]  SumDenOutMin=[]  SumDenOutMax=[]  SumNumOutMin=[]  SumNumOutMax=[]  DivideOutMin=[]  DivideOutMax=[]  UdiffTsProdOutMin=[]  UdiffTsProdOutMax=[]  NTsProdOutMin=[]  NTsProdOutMax=[]  UintegralTsProdOutMin=[]  UintegralTsProdOutMax=[]  UngainTsProdOutMin=[]  UngainTsProdOutMax=[]  IntegratorContinuousStateAttributes=''  IntegratorStateMustResolveToSignalObject=off  IntegratorRTWStateStorageClass=Auto  FilterContinuousStateAttributes=''  FilterStateMustResolveToSignalObject=off  FilterRTWStateStorageClass=Auto  ParallelPVariant=InternalParameters  IdealPVariant=Disabled  IVariant=InternalParameters  DVariant=Disabled  IntegratorVariant=Discrete  SatVariant=Disabled  AWVariant=Passthrough  PCopyVariant=Disabled  TRVariant=Disabled  FdbkBlocksVariant=Forward  IdealPFdbkVariant=Disabled  SatFdbkVariant=Disabled  DerivativeFilterVariant=Disabled  NVariant=Disabled  NCopyVariant=Disabled_SignalSpec  FilterICVariant=Disabled  IntegratorICVariant=InternalICs  ExternalResetVariant=Disabled  TRSumVariant=Passthrough  SumFdbkVariant=Disabled  SumVariant=Sum_PI  TsampFilterVariant=InternalTs  TsampNgainVariant=Passthrough  TsampIntegralVariant=Disabled_SignalSpec  ExternalSaturationOutDataTypeStr=Inherit: Same as second input
  PID Controller2 : slpidlib/PID Controller  Controller=PI  Form=Parallel  TimeDomain=Discrete-time  UseExternalTs=off  SampleTime=5e-4  IntegratorMethod=Forward Euler  FilterMethod=Forward Euler  ControllerParametersSource=internal  P=50  I=400  UseKiTs=off  D=0  N=100  UseFilter=on  TunerSelectOption=Transfer Function Based (PID Tuner App)  InitialConditionSource=internal  InitialConditionForIntegrator=0  InitialConditionForFilter=0  DifferentiatorICPrevScaledInput=0  ExternalReset=none  TrackingMode=off  Kt=1  LimitOutput=off  SatLimitsSource=internal  UpperSaturationLimit=inf  LowerSaturationLimit=-inf  LinearizeAsGain=on  AntiWindupMode=none  Kb=1  LimitIntegrator=off  UpperIntegratorSaturationLimit=inf  LowerIntegratorSaturationLimit=-inf  POutMin=[]  POutMax=[]  IOutMin=[]  IOutMax=[]  DOutMin=[]  DOutMax=[]  NOutMin=[]  NOutMax=[]  SumOutMin=[]  SumOutMax=[]  SaturationOutMin=[]  SaturationOutMax=[]  PParamMin=[]  PParamMax=[]  IParamMin=[]  IParamMax=[]  DParamMin=[]  DParamMax=[]  NParamMin=[]  NParamMax=[]  KbParamMin=[]  KbParamMax=[]  KtParamMin=[]  KtParamMax=[]  KbOutMin=[]  KbOutMax=[]  KtOutMin=[]  KtOutMax=[]  IntegratorOutMin=[]  IntegratorOutMax=[]  FilterOutMin=[]  FilterOutMax=[]  SumI1OutMin=[]  SumI1OutMax=[]  SumI2OutMin=[]  SumI2OutMax=[]  SumI3OutMin=[]  SumI3OutMax=[]  SumI4OutMin=[]  SumI4OutMax=[]  SumDOutMin=[]  SumDOutMax=[]  DifferentiatorOutMin=[]  DifferentiatorOutMax=[]  FilterDiffOutCoefMin=[]  FilterDiffOutCoefMax=[]  ReciprocalOutMin=[]  ReciprocalOutMax=[]  SumDenOutMin=[]  SumDenOutMax=[]  SumNumOutMin=[]  SumNumOutMax=[]  DivideOutMin=[]  DivideOutMax=[]  UdiffTsProdOutMin=[]  UdiffTsProdOutMax=[]  NTsProdOutMin=[]  NTsProdOutMax=[]  UintegralTsProdOutMin=[]  UintegralTsProdOutMax=[]  UngainTsProdOutMin=[]  UngainTsProdOutMax=[]  IntegratorContinuousStateAttributes=''  IntegratorStateMustResolveToSignalObject=off  IntegratorRTWStateStorageClass=Auto  FilterContinuousStateAttributes=''  FilterStateMustResolveToSignalObject=off  FilterRTWStateStorageClass=Auto  ParallelPVariant=InternalParameters  IdealPVariant=Disabled  IVariant=InternalParameters  DVariant=Disabled  IntegratorVariant=Discrete  SatVariant=Disabled  AWVariant=Passthrough  PCopyVariant=Disabled  TRVariant=Disabled  FdbkBlocksVariant=Forward  IdealPFdbkVariant=Disabled  SatFdbkVariant=Disabled  DerivativeFilterVariant=Disabled  NVariant=Disabled  NCopyVariant=Disabled_SignalSpec  FilterICVariant=Disabled  IntegratorICVariant=InternalICs  ExternalResetVariant=Disabled  TRSumVariant=Passthrough  SumFdbkVariant=Disabled  SumVariant=Sum_PI  TsampFilterVariant=InternalTs  TsampNgainVariant=Passthrough  TsampIntegralVariant=Disabled_SignalSpec  ExternalSaturationOutDataTypeStr=Inherit: Same as second input
  PLL (3ph) : spsPLL3phLib/PLL (3ph)  Fmin=59.5  Par_Init=[0, 60]  ParK=[180, 3200, 1]  TcD=1e-4  MaxRateChangeFreq=12  FilterCutOffFreq=25  Ts=1e-5  AGC=on
  Subsystem1 : Subsystem
  Sum1 : Sum  Inputs=|+-
  Sum2 : Sum  Inputs=|+-
  Terminator{,1..4} (5 alike) : Terminator
  WL : Subsystem
  WL1 : Subsystem
  abc to dq0 : spsabctodq0Lib/abc to dq0  Alignment=90 degrees behind phase A axis
  abc to dq1 : spsabctodq0Lib/abc to dq0  Alignment=90 degrees behind phase A axis
  abc to dq2 : spsabctodq0Lib/abc to dq0  Alignment=90 degrees behind phase A axis
  constant : Constant  Value=0
  dq0 to abc : spsdq0toabcLib/dq0 to abc  Alignment=90 degrees behind phase A axis
  Va : Outport  VectorParamsAs1DForOutWhenUnconnected=off
  Vb : Outport  Port=2  VectorParamsAs1DForOutWhenUnconnected=off
  Vc : Outport  Port=3  VectorParamsAs1DForOutWhenUnconnected=off
  wires:
  abc to dq0/1 -> Discrete Transfer Fcn3/1
  PLL (3ph)/2 -> [wt], abc to dq1/2, abc to dq2/2, abc to dq0/2
  Demux1/1 -> Add/1, Subsystem1/3(Ud)
  L1/1 -> WL/3(L), WL1/3(L)
  WL/1(Out1) -> Add/3
  [freq] -> WL1/2(freq), WL/2(freq)
  PLL (3ph)/1 -> [freq]
  Demux2/1 -> Va/1
  Add/1 -> Mux/1
  PID Controller2/1 -> Add1/2
  Demux2/2 -> Vb/1
  WL1/1(Out1) -> Add1/3
  Demux1/2 -> Add1/1
  Add1/1 -> Mux/2
  Mux/1 -> dq0 to abc/1
  Demux2/3 -> Vc/1
  dq0 to abc/1 -> Demux2/1
  Subsystem1/1(Id_ref) -> Sum1/1
  PID Controller1/1 -> Add/2
  [wt] -> dq0 to abc/2
  Subsystem1/2(Iq_ref) -> Sum2/1
  Demux1/3 -> Terminator/1
  Demux/3 -> Terminator1/1
  constant/1 -> Mux/3
  IFabcp/1 -> abc to dq2/1
  abc to dq2/1 -> Discrete Transfer Fcn4/1
  Demux3/3 -> Terminator2/1
  Demux3/2 -> Sum2/2, WL/1(In1)
  Demux3/1 -> Sum1/2, WL1/1(In1)
  Sum1/1 -> PID Controller1/1
  Sum2/1 -> PID Controller2/1
  P_set/1 -> Subsystem1/1(P_ref)
  Q_set/1 -> Subsystem1/2(Q_ref)
  Discrete Transfer Fcn3/1 -> Demux/1
  Discrete Transfer Fcn4/1 -> Demux3/1
  Demux/1 -> Terminator3/1
  Demux/2 -> Terminator4/1
  Discrete Transfer Fcn1/1 -> Demux1/1
  Iabcp/1 -> abc to dq0/1
  Vabcp/1 -> abc to dq1/1, PLL (3ph)/1
  abc to dq1/1 -> Discrete Transfer Fcn1/1

== system IEEE39_IBR_FrequencyControl_Primary_2022b/G5_GFL/PV_PQ3/Freq_Droop ==
  Pref : Inport
  Fref : Inport  Port=2
  Freq : Inport  Port=3
  D : Inport  Port=4
  Divide : Product  Inputs=*/
  Product : Product
  Product1 : Product
  S_base : Constant  Value=Sbase
  Saturation : Saturate  UpperLimit=10*Sbase  LowerLimit=0  ZeroCross=off
  Sum : Sum  Inputs=|+-
  Sum1 : Sum  Inputs=|+-
  Transfer Fcn : TransferFcn  Denominator=[0.318 1]
  Pset : Outport
  wires:
  Freq/1 -> Sum/1
  Fref/1 -> Sum/2, Divide/2
  S_base/1 -> Product/2
  D/1 -> Product1/1
  Product/1 -> Product1/2
  Pref/1 -> Sum1/1
  Product1/1 -> Sum1/2
  Saturation/1 -> Pset/1
  Sum1/1 -> Saturation/1
  Sum/1 -> Divide/1
  Transfer Fcn/1 -> Product/1
  Divide/1 -> Transfer Fcn/1
